simulink model "model4_2"  (R2024a)
settings: Solver=FixedStepAuto  StartTime=0.0  StopTime=36000  FixedStep=0.1  RelTol=1e-3
(part 7 of 7)

== matlab function model4_2/Thermal point/Thermal trans1/Heat Trans ==
  data: Inner_T input; Outer_Heat output; Surrounding_T input; type input
function Outer_Heat = fcn(Inner_T, Surrounding_T, type)
%#codegen
% Inputs
%   Inner_T        : 내부 온도 (scalar)
%   Surrounding    : struct with fields
%       .T         : 주변 온도
%       .mode      : 0 = conduction, 1 = convection

k = 25;    % 열전도도 (W/(m·K)) in-plane
A = 0.01;    % 면적 (m^2)
L = 0.1;    % 길이 (m)
h = 1;    % 대류 열전달계수 (W/(m^2·K))

G_cond = k * A / L;      % 전도 전도도 (W/K)
G_conv = h * A;          % 대류 전도도   (W/K)

if type == 0
    % 전도
    % q = G_cond * (ΔT)
    Outer_Heat = - G_cond * (Inner_T - Surrounding_T);
elseif type == 1
    % 대류
    % q = G_conv * (ΔT)
    Outer_Heat = - G_conv * (Inner_T - Surrounding_T);
else
    % 정의되지 않은 모드일 때
    Outer_Heat = 0;
end

== matlab function model4_2/Thermal point6/Thermal trans1/Heat Trans ==
  data: Inner_T input; Outer_Heat output; Surrounding_T input; type input
function Outer_Heat = fcn(Inner_T, Surrounding_T, type)
%#codegen
% Inputs
%   Inner_T        : 내부 온도 (scalar)
%   Surrounding    : struct with fields
%       .T         : 주변 온도
%       .mode      : 0 = conduction, 1 = convection

k = 25;    % 열전도도 (W/(m·K)) in-plane
A = 0.01;    % 면적 (m^2)
L = 0.1;    % 길이 (m)
h = 1;    % 대류 열전달계수 (W/(m^2·K))

G_cond = k * A / L;      % 전도 전도도 (W/K)
G_conv = h * A;          % 대류 전도도   (W/K)

if type == 0
    % 전도
    % q = G_cond * (ΔT)
    Outer_Heat = - G_cond * (Inner_T - Surrounding_T);
elseif type == 1
    % 대류
    % q = G_conv * (ΔT)
    Outer_Heat = - G_conv * (Inner_T - Surrounding_T);
else
    % 정의되지 않은 모드일 때
    Outer_Heat = 0;
end

== matlab function model4_2/Thermal point6/Thermal trans2/Heat Trans ==
  data: Inner_T input; Outer_Heat output; Surrounding_T input; type input
function Outer_Heat = fcn(Inner_T, Surrounding_T, type)
%#codegen
% Inputs
%   Inner_T        : 내부 온도 (scalar)
%   Surrounding    : struct with fields
%       .T         : 주변 온도
%       .mode      : 0 = conduction, 1 = convection

k = 1;    % 열전도도 (W/(m·K)) through plane
A = 0.01;    % 면적 (m^2)
L = 0.1;    % 길이 (m)
h = 1;    % 대류 열전달계수 (W/(m^2·K))

G_cond = k * A / L;      % 전도 전도도 (W/K)
G_conv = h * A;          % 대류 전도도   (W/K)

if type == 0
    % 전도
    % q = G_cond * (ΔT)
    Outer_Heat = - G_cond * (Inner_T - Surrounding_T);
elseif type == 1
    % 대류
    % q = G_conv * (ΔT)
    Outer_Heat = - G_conv * (Inner_T - Surrounding_T);
else
    % 정의되지 않은 모드일 때
    Outer_Heat = 0;
end

== matlab function model4_2/Thermal point6/Thermal trans3/Heat Trans ==
  data: Inner_T input; Outer_Heat output; Surrounding_T input; type input
function Outer_Heat = fcn(Inner_T, Surrounding_T, type)
%#codegen
% Inputs
%   Inner_T        : 내부 온도 (scalar)
%   Surrounding    : struct with fields
%       .T         : 주변 온도
%       .mode      : 0 = conduction, 1 = convection

k = 1;    % 열전도도 (W/(m·K)) through plane
A = 0.01;    % 면적 (m^2)
L = 0.1;    % 길이 (m)
h = 1;    % 대류 열전달계수 (W/(m^2·K))

G_cond = k * A / L;      % 전도 전도도 (W/K)
G_conv = h * A;          % 대류 전도도   (W/K)

if type == 0
    % 전도
    % q = G_cond * (ΔT)
    Outer_Heat = - G_cond * (Inner_T - Surrounding_T);
elseif type == 1
    % 대류
    % q = G_conv * (ΔT)
    Outer_Heat = - G_conv * (Inner_T - Surrounding_T);
else
    % 정의되지 않은 모드일 때
    Outer_Heat = 0;
end

== matlab function model4_2/Thermal point6/Thermal trans4/Heat Trans ==
  data: Inner_T input; Outer_Heat output; Surrounding_T input; type input
function Outer_Heat = fcn(Inner_T, Surrounding_T, type)
%#codegen
% Inputs
%   Inner_T        : 내부 온도 (scalar)
%   Surrounding    : struct with fields
%       .T         : 주변 온도
%       .mode      : 0 = conduction, 1 = convection

k = 1;    % 열전도도 (W/(m·K)) through plane
A = 0.01;    % 면적 (m^2)
L = 0.1;    % 길이 (m)
h = 1;    % 대류 열전달계수 (W/(m^2·K))

G_cond = k * A / L;      % 전도 전도도 (W/K)
G_conv = h * A;          % 대류 전도도   (W/K)

if type == 0
    % 전도
    % q = G_cond * (ΔT)
    Outer_Heat = - G_cond * (Inner_T - Surrounding_T);
elseif type == 1
    % 대류
    % q = G_conv * (ΔT)
    Outer_Heat = - G_conv * (Inner_T - Surrounding_T);
else
    % 정의되지 않은 모드일 때
    Outer_Heat = 0;
end

== matlab function model4_2/Thermal point6/Thermal trans7/Heat Trans ==
  data: Inner_T input; Outer_Heat output; Surrounding_T input; type input
function Outer_Heat = fcn(Inner_T, Surrounding_T, type)
%#codegen
% Inputs
%   Inner_T        : 내부 온도 (scalar)
%   Surrounding    : struct with fields
%       .T         : 주변 온도
%       .mode      : 0 = conduction, 1 = convection

k = 1;    % 열전도도 (W/(m·K)) through plane
A = 0.01;    % 면적 (m^2)
L = 0.1;    % 길이 (m)
h = 1;    % 대류 열전달계수 (W/(m^2·K))

G_cond = k * A / L;      % 전도 전도도 (W/K)
G_conv = h * A;          % 대류 전도도   (W/K)

if type == 0
    % 전도
    % q = G_cond * (ΔT)
    Outer_Heat = - G_cond * (Inner_T - Surrounding_T);
elseif type == 1
    % 대류
    % q = G_conv * (ΔT)
    Outer_Heat = - G_conv * (Inner_T - Surrounding_T);
else
    % 정의되지 않은 모드일 때
    Outer_Heat = 0;
end

== matlab function model4_2/Thermal point7/Thermal Subsystem/Electrical model/SOC model ==
  data: SOC output; I input; inital_SOC input; capacity input; time_step input
function SOC = fcn(I, inital_SOC, capacity, time_step)
    % Cn = 55.8 * 3600;
    SOC = inital_SOC - (I * time_step / (capacity * 3600));
end

== matlab function model4_2/Thermal point7/Thermal Subsystem/Electrical model/Voltage model ==
  data: R0 input; voltage output; R1 input; R2 input; OCV_Em input; I1 input; I2 input; I input; changed_current_I1 output; changed_current_I2 output; tau1 input; tau2 input; time_step input
function [voltage, changed_current_I1, changed_current_I2] = fcn(R0, R1, R2, OCV_Em, I1, I2, I, tau1, tau2, time_step)
    persistent state_I1 state_I2

    if isempty(state_I1) || isempty(state_I2)
        state_I1 = 0;
        state_I2 = 0;
    else
        state_I1 = I1 * exp(-time_step/tau1) + (1 - exp(-time_step/tau1)) * I;
        state_I2 = I2 * exp(-time_step/tau2) + (1 - exp(-time_step/tau2)) * I;
    end

    voltage = OCV_Em - R0 * I - R1 * state_I1 - R2 * state_I2;
    
    changed_current_I1 = state_I1;
    changed_current_I2 = state_I2;
end

== matlab function model4_2/Thermal point7/Thermal Subsystem/Heat model/Bernardi Equation ==
  data: V input; OCV input; dUdT input; current input; time_step input; T input; totalHeat output
function totalHeat  = fcn(V, OCV, dUdT, current, time_step, T)
    revHeat = current * (T + 273.15) * dUdT;
    irrHeat = current * (OCV - V);
    totalHeat = (-revHeat + irrHeat) * time_step;
end

== matlab function model4_2/Thermal point7/Thermal Subsystem/Heat model/MATLAB Function1 ==
  data: width input; T output; height input; Thickness input; density input; specific_heat input; Inner_heat input; Outer_Heat input; initial_T input
function T = fcn(width, height, Thickness, density, specific_heat, Inner_heat, Outer_Heat, initial_T)
    volume = width * height * Thickness;
    mass = volume * density;
    delta_T = (Inner_heat + Outer_Heat) / (mass * specific_heat);
    T = initial_T + delta_T;
end

== matlab function model4_2/Thermal point/Thermal trans2/Heat Trans ==
  data: Inner_T input; Outer_Heat output; Surrounding_T input; type input
function Outer_Heat = fcn(Inner_T, Surrounding_T, type)
%#codegen
% Inputs
%   Inner_T        : 내부 온도 (scalar)
%   Surrounding    : struct with fields
%       .T         : 주변 온도
%       .mode      : 0 = conduction, 1 = convection

k = 1;    % 열전도도 (W/(m·K)) through plane
A = 0.01;    % 면적 (m^2)
L = 0.1;    % 길이 (m)
h = 1;    % 대류 열전달계수 (W/(m^2·K))

G_cond = k * A / L;      % 전도 전도도 (W/K)
G_conv = h * A;          % 대류 전도도   (W/K)

if type == 0
    % 전도
    % q = G_cond * (ΔT)
    Outer_Heat = - G_cond * (Inner_T - Surrounding_T);
elseif type == 1
    % 대류
    % q = G_conv * (ΔT)
    Outer_Heat = - G_conv * (Inner_T - Surrounding_T);
else
    % 정의되지 않은 모드일 때
    Outer_Heat = 0;
end

== matlab function model4_2/Thermal point7/Thermal trans/Heat Trans ==
  data: Inner_T input; Outer_Heat output; Surrounding_T input; type input
function Outer_Heat = fcn(Inner_T, Surrounding_T, type)
% 물리 상수
k = 25;      % 열전도도 (W/(m·K)) (in-plane)
A = 0.01;    % 면적 (m^2)
L = 0.1;     % 길이 (m)
h = 1;       % 대류 열전달계수 (W/(m^2·K))

% 전도/대류 전도도 계산
G_cond = k * A / L;   % 전도 전도도 (W/K)
G_conv = h * A;       % 대류 전도도   (W/K)

% 열전달 계산
if type == 0
    % 전도
    Outer_Heat = - G_cond * (Inner_T - Surrounding_T);
elseif type == 1
    % 대류
    Outer_Heat = - G_conv * (Inner_T - Surrounding_T);
elseif type == 2
    % 단열 (열전도 없음)
    Outer_Heat = 0;
else
    % 정의되지 않은 모드 → 에러 발생
    error('fcn:InvalidType', 'Unknown heat transfer type: %d', type);
end

== matlab function model4_2/Thermal point7/Thermal trans1/Heat Trans ==
  data: Inner_T input; Outer_Heat output; Surrounding_T input; type input
function Outer_Heat = fcn(Inner_T, Surrounding_T, type)
%#codegen
% Inputs
%   Inner_T        : 내부 온도 (scalar)
%   Surrounding    : struct with fields
%       .T         : 주변 온도
%       .mode      : 0 = conduction, 1 = convection

k = 25;    % 열전도도 (W/(m·K)) in-plane
A = 0.01;    % 면적 (m^2)
L = 0.1;    % 길이 (m)
h = 1;    % 대류 열전달계수 (W/(m^2·K))

G_cond = k * A / L;      % 전도 전도도 (W/K)
G_conv = h * A;          % 대류 전도도   (W/K)

if type == 0
    % 전도
    % q = G_cond * (ΔT)
    Outer_Heat = - G_cond * (Inner_T - Surrounding_T);
elseif type == 1
    % 대류
    % q = G_conv * (ΔT)
    Outer_Heat = - G_conv * (Inner_T - Surrounding_T);
else
    % 정의되지 않은 모드일 때
    Outer_Heat = 0;
end

== matlab function model4_2/Thermal point7/Thermal trans2/Heat Trans ==
  data: Inner_T input; Outer_Heat output; Surrounding_T input; type input
function Outer_Heat = fcn(Inner_T, Surrounding_T, type)
%#codegen
% Inputs
%   Inner_T        : 내부 온도 (scalar)
%   Surrounding    : struct with fields
%       .T         : 주변 온도
%       .mode      : 0 = conduction, 1 = convection

k = 1;    % 열전도도 (W/(m·K)) through plane
A = 0.01;    % 면적 (m^2)
L = 0.1;    % 길이 (m)
h = 1;    % 대류 열전달계수 (W/(m^2·K))

G_cond = k * A / L;      % 전도 전도도 (W/K)
G_conv = h * A;          % 대류 전도도   (W/K)

if type == 0
    % 전도
    % q = G_cond * (ΔT)
    Outer_Heat = - G_cond * (Inner_T - Surrounding_T);
elseif type == 1
    % 대류
    % q = G_conv * (ΔT)
    Outer_Heat = - G_conv * (Inner_T - Surrounding_T);
else
    % 정의되지 않은 모드일 때
    Outer_Heat = 0;
end

== matlab function model4_2/Thermal point7/Thermal trans3/Heat Trans ==
  data: Inner_T input; Outer_Heat output; Surrounding_T input; type input
function Outer_Heat = fcn(Inner_T, Surrounding_T, type)
%#codegen
% Inputs
%   Inner_T        : 내부 온도 (scalar)
%   Surrounding    : struct with fields
%       .T         : 주변 온도
%       .mode      : 0 = conduction, 1 = convection

k = 1;    % 열전도도 (W/(m·K)) through plane
A = 0.01;    % 면적 (m^2)
L = 0.1;    % 길이 (m)
h = 1;    % 대류 열전달계수 (W/(m^2·K))

G_cond = k * A / L;      % 전도 전도도 (W/K)
G_conv = h * A;          % 대류 전도도   (W/K)

if type == 0
    % 전도
    % q = G_cond * (ΔT)
    Outer_Heat = - G_cond * (Inner_T - Surrounding_T);
elseif type == 1
    % 대류
    % q = G_conv * (ΔT)
    Outer_Heat = - G_conv * (Inner_T - Surrounding_T);
else
    % 정의되지 않은 모드일 때
    Outer_Heat = 0;
end

== matlab function model4_2/Thermal point7/Thermal trans4/Heat Trans ==
  data: Inner_T input; Outer_Heat output; Surrounding_T input; type input
function Outer_Heat = fcn(Inner_T, Surrounding_T, type)
%#codegen
% Inputs
%   Inner_T        : 내부 온도 (scalar)
%   Surrounding    : struct with fields
%       .T         : 주변 온도
%       .mode      : 0 = conduction, 1 = convection

k = 1;    % 열전도도 (W/(m·K)) through plane
A = 0.01;    % 면적 (m^2)
L = 0.1;    % 길이 (m)
h = 1;    % 대류 열전달계수 (W/(m^2·K))

G_cond = k * A / L;      % 전도 전도도 (W/K)
G_conv = h * A;          % 대류 전도도   (W/K)

if type == 0
    % 전도
    % q = G_cond * (ΔT)
    Outer_Heat = - G_cond * (Inner_T - Surrounding_T);
elseif type == 1
    % 대류
    % q = G_conv * (ΔT)
    Outer_Heat = - G_conv * (Inner_T - Surrounding_T);
else
    % 정의되지 않은 모드일 때
    Outer_Heat = 0;
end

== matlab function model4_2/Thermal point7/Thermal trans7/Heat Trans ==
  data: Inner_T input; Outer_Heat output; Surrounding_T input; type input
function Outer_Heat = fcn(Inner_T, Surrounding_T, type)
%#codegen
% Inputs
%   Inner_T        : 내부 온도 (scalar)
%   Surrounding    : struct with fields
%       .T         : 주변 온도
%       .mode      : 0 = conduction, 1 = convection

k = 1;    % 열전도도 (W/(m·K)) through plane
A = 0.01;    % 면적 (m^2)
L = 0.1;    % 길이 (m)
h = 1;    % 대류 열전달계수 (W/(m^2·K))

G_cond = k * A / L;      % 전도 전도도 (W/K)
G_conv = h * A;          % 대류 전도도   (W/K)

if type == 0
    % 전도
    % q = G_cond * (ΔT)
    Outer_Heat = - G_cond * (Inner_T - Surrounding_T);
elseif type == 1
    % 대류
    % q = G_conv * (ΔT)
    Outer_Heat = - G_conv * (Inner_T - Surrounding_T);
else
    % 정의되지 않은 모드일 때
    Outer_Heat = 0;
end

== matlab function model4_2/Thermal point8/Thermal Subsystem/Electrical model/SOC model ==
  data: SOC output; I input; inital_SOC input; capacity input; time_step input
function SOC = fcn(I, inital_SOC, capacity, time_step)
    % Cn = 55.8 * 3600;
    SOC = inital_SOC - (I * time_step / (capacity * 3600));
end

== matlab function model4_2/Thermal point8/Thermal Subsystem/Electrical model/Voltage model ==
  data: R0 input; voltage output; R1 input; R2 input; OCV_Em input; I1 input; I2 input; I input; changed_current_I1 output; changed_current_I2 output; tau1 input; tau2 input; time_step input
function [voltage, changed_current_I1, changed_current_I2] = fcn(R0, R1, R2, OCV_Em, I1, I2, I, tau1, tau2, time_step)
    persistent state_I1 state_I2

    if isempty(state_I1) || isempty(state_I2)
        state_I1 = 0;
        state_I2 = 0;
    else
        state_I1 = I1 * exp(-time_step/tau1) + (1 - exp(-time_step/tau1)) * I;
        state_I2 = I2 * exp(-time_step/tau2) + (1 - exp(-time_step/tau2)) * I;
    end

    voltage = OCV_Em - R0 * I - R1 * state_I1 - R2 * state_I2;
    
    changed_current_I1 = state_I1;
    changed_current_I2 = state_I2;
end

== matlab function model4_2/Thermal point/Thermal trans3/Heat Trans ==
  data: Inner_T input; Outer_Heat output; Surrounding_T input; type input
function Outer_Heat = fcn(Inner_T, Surrounding_T, type)
%#codegen
% Inputs
%   Inner_T        : 내부 온도 (scalar)
%   Surrounding    : struct with fields
%       .T         : 주변 온도
%       .mode      : 0 = conduction, 1 = convection

k = 1;    % 열전도도 (W/(m·K)) through plane
A = 0.01;    % 면적 (m^2)
L = 0.1;    % 길이 (m)
h = 1;    % 대류 열전달계수 (W/(m^2·K))

G_cond = k * A / L;      % 전도 전도도 (W/K)
G_conv = h * A;          % 대류 전도도   (W/K)

if type == 0
    % 전도
    % q = G_cond * (ΔT)
    Outer_Heat = - G_cond * (Inner_T - Surrounding_T);
elseif type == 1
    % 대류
    % q = G_conv * (ΔT)
    Outer_Heat = - G_conv * (Inner_T - Surrounding_T);
else
    % 정의되지 않은 모드일 때
    Outer_Heat = 0;
end

== matlab function model4_2/Thermal point8/Thermal Subsystem/Heat model/Bernardi Equation ==
  data: V input; OCV input; dUdT input; current input; time_step input; T input; totalHeat output
function totalHeat  = fcn(V, OCV, dUdT, current, time_step, T)
    revHeat = current * (T + 273.15) * dUdT;
    irrHeat = current * (OCV - V);
    totalHeat = (-revHeat + irrHeat) * time_step;
end

== matlab function model4_2/Thermal point8/Thermal Subsystem/Heat model/MATLAB Function1 ==
  data: width input; T output; height input; Thickness input; density input; specific_heat input; Inner_heat input; Outer_Heat input; initial_T input
function T = fcn(width, height, Thickness, density, specific_heat, Inner_heat, Outer_Heat, initial_T)
    volume = width * height * Thickness;
    mass = volume * density;
    delta_T = (Inner_heat + Outer_Heat) / (mass * specific_heat);
    T = initial_T + delta_T;
end

== matlab function model4_2/Thermal point8/Thermal trans/Heat Trans ==
  data: Inner_T input; Outer_Heat output; Surrounding_T input; type input
function Outer_Heat = fcn(Inner_T, Surrounding_T, type)
% 물리 상수
k = 25;      % 열전도도 (W/(m·K)) (in-plane)
A = 0.01;    % 면적 (m^2)
L = 0.1;     % 길이 (m)
h = 1;       % 대류 열전달계수 (W/(m^2·K))

% 전도/대류 전도도 계산
G_cond = k * A / L;   % 전도 전도도 (W/K)
G_conv = h * A;       % 대류 전도도   (W/K)

% 열전달 계산
if type == 0
    % 전도
    Outer_Heat = - G_cond * (Inner_T - Surrounding_T);
elseif type == 1
    % 대류
    Outer_Heat = - G_conv * (Inner_T - Surrounding_T);
elseif type == 2
    % 단열 (열전도 없음)
    Outer_Heat = 0;
else
    % 정의되지 않은 모드 → 에러 발생
    error('fcn:InvalidType', 'Unknown heat transfer type: %d', type);
end

== matlab function model4_2/Thermal point8/Thermal trans1/Heat Trans ==
  data: Inner_T input; Outer_Heat output; Surrounding_T input; type input
function Outer_Heat = fcn(Inner_T, Surrounding_T, type)
%#codegen
% Inputs
%   Inner_T        : 내부 온도 (scalar)
%   Surrounding    : struct with fields
%       .T         : 주변 온도
%       .mode      : 0 = conduction, 1 = convection

k = 25;    % 열전도도 (W/(m·K)) in-plane
A = 0.01;    % 면적 (m^2)
L = 0.1;    % 길이 (m)
h = 1;    % 대류 열전달계수 (W/(m^2·K))

G_cond = k * A / L;      % 전도 전도도 (W/K)
G_conv = h * A;          % 대류 전도도   (W/K)

if type == 0
    % 전도
    % q = G_cond * (ΔT)
    Outer_Heat = - G_cond * (Inner_T - Surrounding_T);
elseif type == 1
    % 대류
    % q = G_conv * (ΔT)
    Outer_Heat = - G_conv * (Inner_T - Surrounding_T);
else
    % 정의되지 않은 모드일 때
    Outer_Heat = 0;
end

== matlab function model4_2/Thermal point8/Thermal trans2/Heat Trans ==
  data: Inner_T input; Outer_Heat output; Surrounding_T input; type input
function Outer_Heat = fcn(Inner_T, Surrounding_T, type)
%#codegen
% Inputs
%   Inner_T        : 내부 온도 (scalar)
%   Surrounding    : struct with fields
%       .T         : 주변 온도
%       .mode      : 0 = conduction, 1 = convection

k = 1;    % 열전도도 (W/(m·K)) through plane
A = 0.01;    % 면적 (m^2)
L = 0.1;    % 길이 (m)
h = 1;    % 대류 열전달계수 (W/(m^2·K))

G_cond = k * A / L;      % 전도 전도도 (W/K)
G_conv = h * A;          % 대류 전도도   (W/K)

if type == 0
    % 전도
    % q = G_cond * (ΔT)
    Outer_Heat = - G_cond * (Inner_T - Surrounding_T);
elseif type == 1
    % 대류
    % q = G_conv * (ΔT)
    Outer_Heat = - G_conv * (Inner_T - Surrounding_T);
else
    % 정의되지 않은 모드일 때
    Outer_Heat = 0;
end

== matlab function model4_2/Thermal point8/Thermal trans3/Heat Trans ==
  data: Inner_T input; Outer_Heat output; Surrounding_T input; type input
function Outer_Heat = fcn(Inner_T, Surrounding_T, type)
%#codegen
% Inputs
%   Inner_T        : 내부 온도 (scalar)
%   Surrounding    : struct with fields
%       .T         : 주변 온도
%       .mode      : 0 = conduction, 1 = convection

k = 1;    % 열전도도 (W/(m·K)) through plane
A = 0.01;    % 면적 (m^2)
L = 0.1;    % 길이 (m)
h = 1;    % 대류 열전달계수 (W/(m^2·K))

G_cond = k * A / L;      % 전도 전도도 (W/K)
G_conv = h * A;          % 대류 전도도   (W/K)

if type == 0
    % 전도
    % q = G_cond * (ΔT)
    Outer_Heat = - G_cond * (Inner_T - Surrounding_T);
elseif type == 1
    % 대류
    % q = G_conv * (ΔT)
    Outer_Heat = - G_conv * (Inner_T - Surrounding_T);
else
    % 정의되지 않은 모드일 때
    Outer_Heat = 0;
end

== matlab function model4_2/Thermal point8/Thermal trans4/Heat Trans ==
  data: Inner_T input; Outer_Heat output; Surrounding_T input; type input
function Outer_Heat = fcn(Inner_T, Surrounding_T, type)
%#codegen
% Inputs
%   Inner_T        : 내부 온도 (scalar)
%   Surrounding    : struct with fields
%       .T         : 주변 온도
%       .mode      : 0 = conduction, 1 = convection

k = 1;    % 열전도도 (W/(m·K)) through plane
A = 0.01;    % 면적 (m^2)
L = 0.1;    % 길이 (m)
h = 1;    % 대류 열전달계수 (W/(m^2·K))

G_cond = k * A / L;      % 전도 전도도 (W/K)
G_conv = h * A;          % 대류 전도도   (W/K)

if type == 0
    % 전도
    % q = G_cond * (ΔT)
    Outer_Heat = - G_cond * (Inner_T - Surrounding_T);
elseif type == 1
    % 대류
    % q = G_conv * (ΔT)
    Outer_Heat = - G_conv * (Inner_T - Surrounding_T);
else
    % 정의되지 않은 모드일 때
    Outer_Heat = 0;
end

== matlab function model4_2/Thermal point8/Thermal trans7/Heat Trans ==
  data: Inner_T input; Outer_Heat output; Surrounding_T input; type input
function Outer_Heat = fcn(Inner_T, Surrounding_T, type)
%#codegen
% Inputs
%   Inner_T        : 내부 온도 (scalar)
%   Surrounding    : struct with fields
%       .T         : 주변 온도
%       .mode      : 0 = conduction, 1 = convection

k = 1;    % 열전도도 (W/(m·K)) through plane
A = 0.01;    % 면적 (m^2)
L = 0.1;    % 길이 (m)
h = 1;    % 대류 열전달계수 (W/(m^2·K))

G_cond = k * A / L;      % 전도 전도도 (W/K)
G_conv = h * A;          % 대류 전도도   (W/K)

if type == 0
    % 전도
    % q = G_cond * (ΔT)
    Outer_Heat = - G_cond * (Inner_T - Surrounding_T);
elseif type == 1
    % 대류
    % q = G_conv * (ΔT)
    Outer_Heat = - G_conv * (Inner_T - Surrounding_T);
else
    % 정의되지 않은 모드일 때
    Outer_Heat = 0;
end

== matlab function model4_2/Thermal point9/Thermal Subsystem/Electrical model/SOC model ==
  data: SOC output; I input; inital_SOC input; capacity input; time_step input
function SOC = fcn(I, inital_SOC, capacity, time_step)
    % Cn = 55.8 * 3600;
    SOC = inital_SOC - (I * time_step / (capacity * 3600));
end
